simulink model "zumo_plant_custom_heading_original"  (R2014b)
settings: Solver=ode3  SolverMode=SingleTasking  StartTime=0.0  StopTime=2  FixedStep=0.01  RelTol=1e-3
PreLoadFcn:
  | evalin('base','sim=1;');
  | prepareCurrentFolderForZumo;
  | load MagnetometerBus;
model workspace (MAT data in the model file):
  axleLength = Simulink.Parameter
  axleLength.Value = 9.8
  axleLength.Description = 'Distance between tire contact points
    | of the two wheels/treads
    | in units of centimeters.'
  axleLength.DataType = 'auto'
  commandPercmPerSecond = Simulink.Parameter
  commandPercmPerSecond.Value = 3.9547
  commandPercmPerSecond.Description = 'Convert units of ''command'' 
    | to units of ''cm/s''.
    | 
    | ''command'' is a value in the range [-256, 255].'
  commandPercmPerSecond.DataType = 'auto'
  symmetrizeMotors = Simulink.Parameter
  symmetrizeMotors.Value = 1
  symmetrizeMotors.Description = 'Scale one of the motor commands down 
    | (not up) to balance the motors. 
    | Once balanced, a value of x sent to either
    | motor will produce the same rate of rotation
    | in both motors.'
  symmetrizeMotors.DataType = 'auto'
  sampleTime = Simulink.Parameter
  sampleTime.Value = 0.01
  sampleTime.Description = 'Sample time (in seconds) of the trajectory simulator.'
  sampleTime.DataType = 'auto'
  commandThreshold = Simulink.Parameter
  commandThreshold.Value = 31.875
  commandThreshold.DataType = 'auto'
  lineThreshold = Simulink.Parameter
  lineThreshold.Value = 500
  lineThreshold.DataType = 'auto'
  velocity = Simulink.Parameter
  velocity.Value = 10
  velocity.Description = 'cm / s'
  velocity.DataType = 'auto'
  waveLength = Simulink.Parameter
  waveLength.Value = 8.6
  waveLength.Description = 'Units of cm.
    | 
    | The following condition must be satisfied: 
    | waveLength > 2*pi * velocity / sqrt(0.5 / sampleTime)
    | 
    | For reference,
    | robotLength = 8.6 cm
    | '
  waveLength.DataType = 'auto'
  compassBias = Simulink.Parameter
  compassBias.Value = 0
  compassBias.DataType = 'auto'
undefined symbols (not defined in the file or in its folder): magnitude
libraries: simulink x5, ZumoBotLib x2
settings Model: ExtModeTrigDuration=2  Creator=pkasseba  LastModifiedBy=sandip
settings OptimizationCC: OptimizeModelRefInitCode=on  LifeSpan=1
settings DebuggingCC: UnderspecifiedInitializationDetection=Classic  MergeDetectMultiDrivingBlocksExec=none  SolverPrmCheckMsg=none  StateNameClashWarn=warning
settings HardwareCC: ProdBitPerInt=16  ProdBitPerPointer=8  ProdIntDivRoundTo=Zero  ProdEndianess=LittleEndian  ProdWordSize=8  ProdHWDeviceType=Atmel->AVR
settings SFSimCC: SimParseCustomCode=off
settings RTWCC: SystemTargetFile=realtime.tlc  GenerateMakefile=off  TemplateMakefile=realtime.tmf  Description=Run on Target Hardware  RTWVerbose=off  ProcessScript=realtime_make_rtw_hook
settings STFCustomTargetCC: TargetLibSuffix=.a  GenerateSampleERTMain=on  ERTCustomFileBanners=on  SupportNonInlinedSFcns=off  SupportVariableSizeSignals=on  MATLABClassNameForMDSCustomization=Simulink.SoftwareTarget.ERTCustomization  GRTInterface=off  SystemTargetFile=realtime.tlc
settings ERTTargetCC: GenerateSampleERTMain=on  ParMdlRefBuildCompliant=off  CompOptLevelCompliant=off  ConcurrentExecutionCompliant=off  CombineOutputUpdateFcns=off  ERTFirstTimeCompliant=off  SupportContinuousTime=on  SupportVariableSizeSignals=on  ModelStepFunctionPrototypeControlCompliant=off  CPPClassGenCompliant=off  ExtModeTransport=3  ExtModeMexFile=ext_serial_win32_comm  ExtModeMexArgs=0 1 9600  InlinedParameterPlacement=NonHierarchical  ERTSrcFileBannerTemplate=realtime_code_template.cgt  ERTHdrFileBannerTemplate=realtime_code_template.cgt  ERTDataSrcFileTemplate=realtime_code_template.cgt  ERTDataHdrFileTemplate=realtime_code_template.cgt  ERTCustomFileTemplate=realtime_file_process.tlc

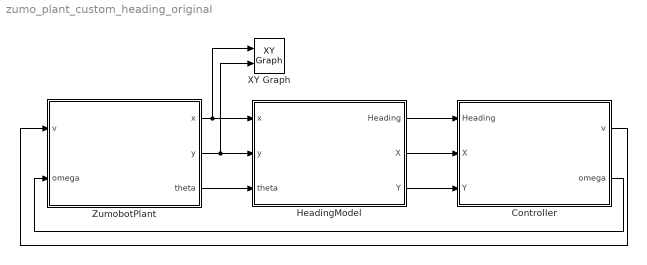
== system zumo_plant_custom_heading_original ==
  Controller : Subsystem
  HeadingModel : Subsystem  Variant=on
  XY Graph : simulink/Sinks/XY Graph  xmin=-10  xmax=50  ymin=-10  ymax=50  st=-1
  ZumobotPlant : Subsystem  Variant=on
  wires:
  Controller/1(v) -> ZumobotPlant/1(v)
  ZumobotPlant/1(x) -> XY Graph/1, HeadingModel/1(x)
  ZumobotPlant/2(y) -> XY Graph/2, HeadingModel/2(y)
  HeadingModel/1(Heading) -> Controller/1(Heading)
  Controller/2(omega) -> ZumobotPlant/2(omega)
  ZumobotPlant/3(theta) -> HeadingModel/3(theta)
  HeadingModel/2(X) -> Controller/2(X)
  HeadingModel/3(Y) -> Controller/3(Y)

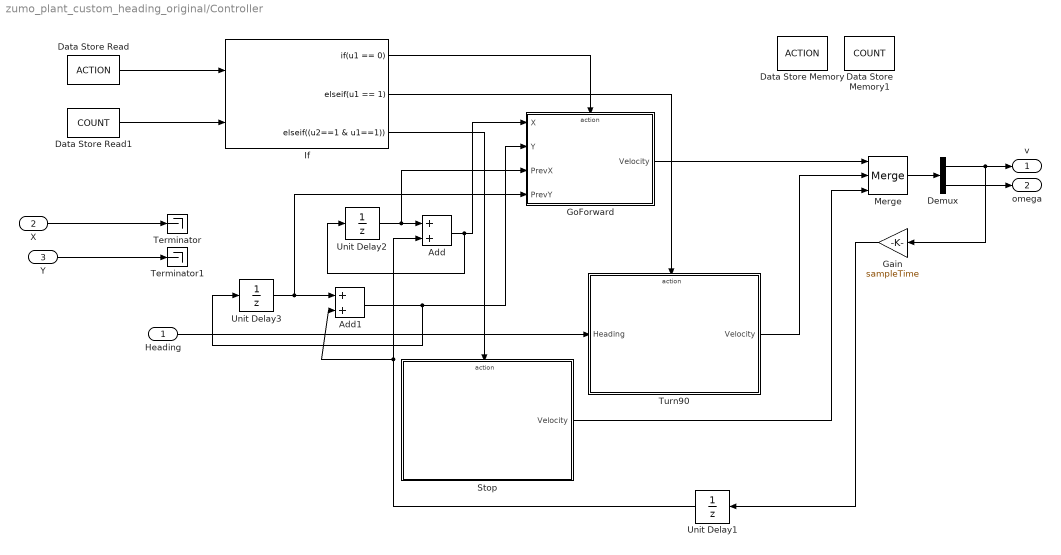
== system zumo_plant_custom_heading_original/Controller ==
  Heading : Inport
  X : Inport  Port=2
  Y : Inport  Port=3
  Add : Sum
  Add1 : Sum
  Data Store Memory : DataStoreMemory  DataStoreName=ACTION  ReadBeforeWriteMsg=warning  WriteAfterWriteMsg=warning  WriteAfterReadMsg=warning
  Data Store Memory1 : DataStoreMemory  DataStoreName=COUNT  ReadBeforeWriteMsg=warning  WriteAfterWriteMsg=warning  WriteAfterReadMsg=warning
  Data Store Read : DataStoreRead  DataStoreName=ACTION  SampleTime=sampleTime
  Data Store Read1 : DataStoreRead  DataStoreName=COUNT  SampleTime=sampleTime
  Demux : Demux  Outputs=2
  Gain : Gain  Gain=sampleTime
  GoForward : Subsystem  TreatAsAtomicUnit=on
  If : If  NumInputs=2  IfExpression=u1 == 0  ElseIfExpressions=u1 == 1, (u2==1 & u1==1)  ShowElse=off
  Merge : Merge  Inputs=3  InitialOutput=[0,0]
  Stop : Subsystem  TreatAsAtomicUnit=on
  Terminator : Terminator
  Terminator1 : Terminator
  Turn90 : Subsystem  TreatAsAtomicUnit=on
  Unit Delay1 : UnitDelay  SampleTime=-1
  Unit Delay2 : UnitDelay  SampleTime=-1
  Unit Delay3 : UnitDelay  SampleTime=-1
  v : Outport
  omega : Outport  Port=2
  wires:
  Demux/1 -> Gain/1, v/1
  Data Store Read/1 -> If/1
  If/1 -> GoForward/Action
  Heading/1 -> Turn90/1(Heading)
  If/2 -> Turn90/Action
  Data Store Read1/1 -> If/2
  If/3 -> Stop/Action
  GoForward/1(Velocity) -> Merge/1
  Turn90/1(Velocity) -> Merge/2
  Stop/1(Velocity) -> Merge/3
  Merge/1 -> Demux/1
  Demux/2 -> omega/1
  Gain/1 -> Unit Delay1/1
  Unit Delay2/1 -> GoForward/3(PrevX), Add/1
  Add/1 -> Unit Delay2/1, GoForward/1(X)
  Unit Delay3/1 -> GoForward/4(PrevY), Add1/1
  Add1/1 -> Unit Delay3/1, GoForward/2(Y)
  X/1 -> Terminator/1
  Y/1 -> Terminator1/1
  Unit Delay1/1 -> Add1/2, Add/2

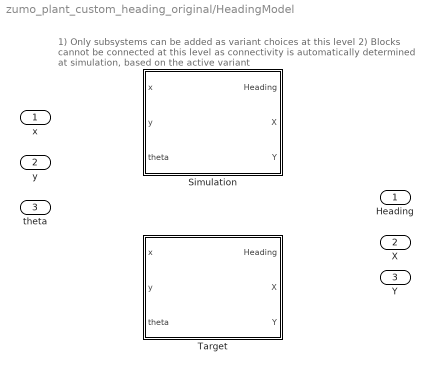
== system zumo_plant_custom_heading_original/HeadingModel ==
  note: 1) Only subsystems can be added as variant choices at this level
      | 2) Blocks cannot be connected at this level as connectivity is
      | automatically determined at simulation, based on the active variant
  x : Inport
  y : Inport  Port=2
  theta : Inport  Port=3
  Simulation : Subsystem  VariantControl=sim==1
  Target : Subsystem  VariantControl=sim==0
  Heading : Outport
  X : Outport  Port=2
  Y : Outport  Port=3

== system zumo_plant_custom_heading_original/ZumobotPlant ==
  note: 1) Only subsystems can be added as variant choices at this level
      | 2) Blocks cannot be connected at this level as connectivity is
      | automatically determined at simulation, based on the active variant
  v : Inport
  omega : Inport  Port=2
  Simulation : Subsystem  VariantControl=sim==1
  Target : Subsystem  VariantControl=sim==0
  x : Outport
  y : Outport  Port=2
  theta : Outport  Port=3

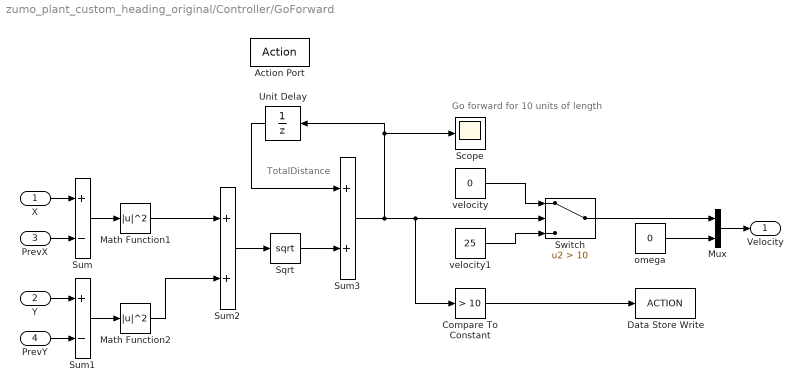
== system zumo_plant_custom_heading_original/Controller/GoForward ==
  note: Go forward for 10 units of length
  note: TotalDistance
  X : Inport
  Y : Inport  Port=2
  PrevX : Inport  Port=3
  PrevY : Inport  Port=4
  Action Port : ActionPort  InitializeStates=reset  ActionType=then
  Compare To Constant : simulink/Logic and Bit Operations/Compare To Constant  relop=>  const=10  OutDataTypeStr=boolean
  Data Store Write : DataStoreWrite  DataStoreName=ACTION
  Math Function1 : Math  Operator=magnitude^2  SaturateOnIntegerOverflow=on
  Math Function2 : Math  Operator=magnitude^2  SaturateOnIntegerOverflow=on
  Mux : Mux  Inputs=2
  Scope : Scope
      settings: YMin=0  YMax=50
  Sqrt : Sqrt  SaturateOnIntegerOverflow=on
  Sum : Sum  Inputs=+-
  Sum1 : Sum  Inputs=+-
  Sum2 : Sum
  Sum3 : Sum
  Switch : Switch  Criteria=u2 > Threshold  Threshold=10
  Unit Delay : UnitDelay  SampleTime=-1
  omega : Constant  Value=0
  velocity : Constant  Value=0
  velocity1 : Constant  Value=25
  Velocity : Outport  InitialOutput=[0 0]
  wires:
  X/1 -> Sum/1
  PrevX/1 -> Sum/2
  Y/1 -> Sum1/1
  PrevY/1 -> Sum1/2
  Sum/1 -> Math Function1/1
  Sum1/1 -> Math Function2/1
  Sum2/1 -> Sqrt/1
  Math Function2/1 -> Sum2/2
  Math Function1/1 -> Sum2/1
  Sqrt/1 -> Sum3/2
  Unit Delay/1 -> Sum3/1
  Mux/1 -> Velocity/1
  velocity/1 -> Switch/1
  velocity1/1 -> Switch/3
  Switch/1 -> Mux/1
  omega/1 -> Mux/2
  Compare To Constant/1 -> Data Store Write/1
  Sum3/1 -> Scope/1, Unit Delay/1, Compare To Constant/1, Switch/2

== system zumo_plant_custom_heading_original/Controller/Stop ==
  Action Port : ActionPort  InitializeStates=reset  ActionType=elseif
  Mux : Mux  Inputs=2
  omega : Constant  Value=0
  speed : Constant  Value=0
  Velocity : Outport  InitialOutput=[ 0 0 ]
  wires:
  Mux/1 -> Velocity/1
  speed/1 -> Mux/1
  omega/1 -> Mux/2

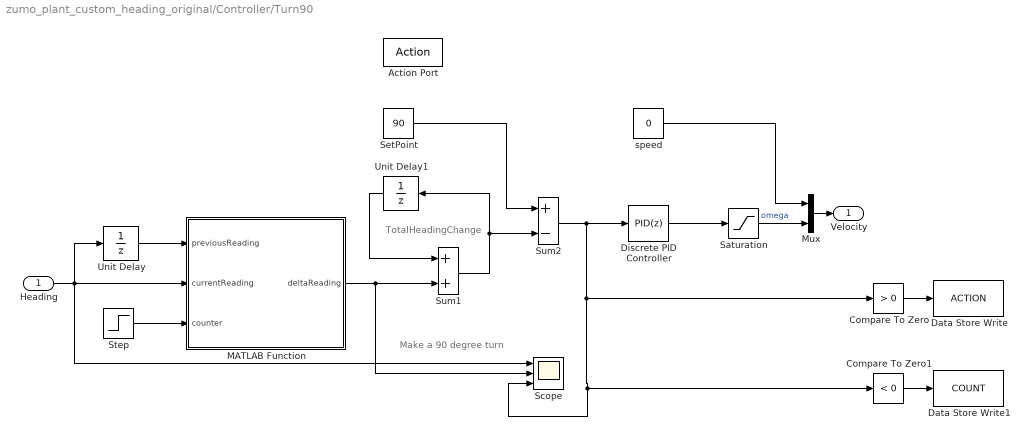
== system zumo_plant_custom_heading_original/Controller/Turn90 ==
  note: Make a 90 degree turn
  note: TotalHeadingChange
  Heading : Inport
  Action Port : ActionPort  InitializeStates=reset  ActionType=elseif
  Compare To Zero : simulink/Logic and Bit Operations/Compare To Zero  relop=>  OutDataTypeStr=boolean
  Compare To Zero1 : simulink/Logic and Bit Operations/Compare To Zero  relop=<  OutDataTypeStr=boolean
  Data Store Write : DataStoreWrite  DataStoreName=ACTION
  Data Store Write1 : DataStoreWrite  DataStoreName=COUNT
  Discrete PID Controller : simulink/Continuous/PID Controller  Controller=PID  TimeDomain=Discrete-time  SampleTime=0.01  IntegratorMethod=Forward Euler  FilterMethod=Forward Euler  Form=Parallel  P=100  I=0  D=0  N=100  InitialConditionSource=internal  InitialConditionForIntegrator=0  InitialConditionForFilter=0  ExternalReset=none  LimitOutput=off  UpperSaturationLimit=inf  LowerSaturationLimit=-inf  LinearizeAsGain=off  AntiWindupMode=none  Kb=1  TrackingMode=off  Kt=1  PParamMin=[]  PParamMax=[]  IParamMin=[]  IParamMax=[]  DParamMin=[]  DParamMax=[]  NParamMin=[]  NParamMax=[]  KbParamMin=[]  KbParamMax=[]  KtParamMin=[]  KtParamMax=[]  POutMin=[]  POutMax=[]  IOutMin=[]  IOutMax=[]  DOutMin=[]  DOutMax=[]  NOutMin=[]  NOutMax=[]  KbOutMin=[]  KbOutMax=[]  KtOutMin=[]  KtOutMax=[]  IntegratorOutMin=[]  IntegratorOutMax=[]  FilterOutMin=[]  FilterOutMax=[]  SumOutMin=[]  SumOutMax=[]  SumI1OutMin=[]  SumI1OutMax=[]  SumI2OutMin=[]  SumI2OutMax=[]  SumI3OutMin=[]  SumI3OutMax=[]  SumDOutMin=[]  SumDOutMax=[]  SaturationOutMin=[]  SaturationOutMax=[]  IntegratorContinuousStateAttributes=''  IntegratorStateMustResolveToSignalObject=off  IntegratorRTWStateStorageClass=Auto  FilterContinuousStateAttributes=''  FilterStateMustResolveToSignalObject=off  FilterRTWStateStorageClass=Auto  DifferentiatorICPrevScaledInput=0  DifferentiatorOutMin=[]  DifferentiatorOutMax=[]  UseFilter=on
  MATLAB Function : MATLAB Function  TreatAsAtomicUnit=on
  Mux : Mux  Inputs=2
  Saturation : Saturate  UpperLimit=200  LowerLimit=0
  Scope : Scope  NumInputPorts=3
      settings: YMin=252.7~-1~-4.2  YMax=279.3~1~-3.8
  SetPoint : Constant  Value=90
  Step : Step  Time=2*sampleTime  SampleTime=sampleTime
  Sum1 : Sum
  Sum2 : Sum  Inputs=+-
  Unit Delay : UnitDelay  SampleTime=-1
  Unit Delay1 : UnitDelay  SampleTime=-1
  speed : Constant  Value=0
  Velocity : Outport  InitialOutput=[0 0]
  wires:
  Sum2/1 -> Discrete PID Controller/1, Scope/3, Compare To Zero1/1, Compare To Zero/1
  Saturation/1 -> Mux/2  "omega"
  Sum1/1 -> Unit Delay1/1, Sum2/2
  MATLAB Function/1(deltaReading) -> Scope/2, Sum1/2
  SetPoint/1 -> Sum2/1
  Step/1 -> MATLAB Function/3(counter)
  Unit Delay/1 -> MATLAB Function/1(previousReading)
  Heading/1 -> Unit Delay/1, MATLAB Function/2(currentReading), Scope/1
  Unit Delay1/1 -> Sum1/1
  Mux/1 -> Velocity/1
  speed/1 -> Mux/1
  Compare To Zero/1 -> Data Store Write/1
  Compare To Zero1/1 -> Data Store Write1/1
  Discrete PID Controller/1 -> Saturation/1

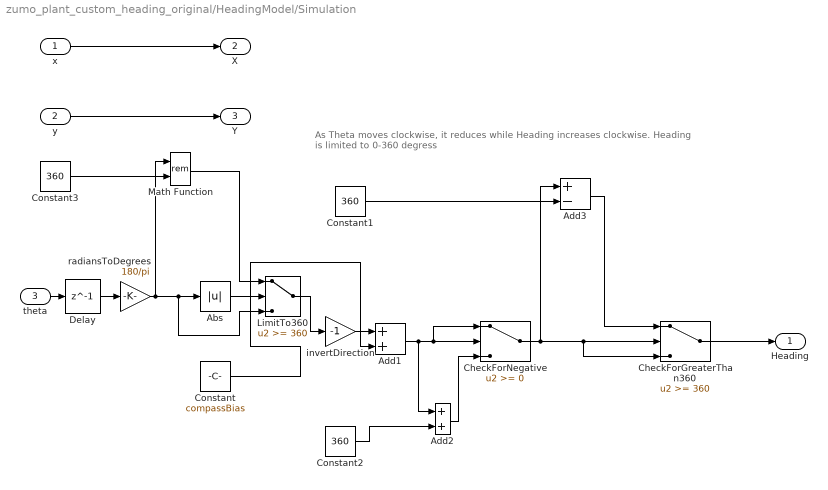
== system zumo_plant_custom_heading_original/HeadingModel/Simulation ==
  note: As Theta moves clockwise, it reduces while Heading increases clockwise.
      | Heading is limited to 0-360 degress
  x : Inport
  y : Inport  Port=2
  theta : Inport  Port=3
  Abs : Abs
  Add1 : Sum
  Add2 : Sum
  Add3 : Sum  Inputs=+-
  CheckForGreaterThan360 : Switch  Threshold=360
  CheckForNegative : Switch
  Constant : Constant  Value=compassBias
  Constant1 : Constant  Value=360
  Constant2 : Constant  Value=360
  Constant3 : Constant  Value=360
  Delay : Delay  DelayLength=1  InitialCondition=2*pi  SampleTime=sampleTime
  LimitTo360 : Switch  Threshold=360
  Math Function : Math  Operator=rem  SaturateOnIntegerOverflow=on
  invertDirection : Gain  Gain=-1
  radiansToDegrees : Gain  Gain=180/pi
  Heading : Outport
  X : Outport  Port=2
  Y : Outport  Port=3
  wires:
  x/1 -> X/1
  y/1 -> Y/1
  theta/1 -> Delay/1
  Delay/1 -> radiansToDegrees/1
  Constant/1 -> Add1/2
  Constant1/1 -> Add3/2
  CheckForGreaterThan360/1 -> Heading/1
  Add3/1 -> CheckForGreaterThan360/1
  invertDirection/1 -> Add1/1
  Add1/1 -> Add2/1, CheckForNegative/2, CheckForNegative/1
  CheckForNegative/1 -> CheckForGreaterThan360/3, CheckForGreaterThan360/2, Add3/1
  Constant2/1 -> Add2/2
  Add2/1 -> CheckForNegative/3
  radiansToDegrees/1 -> Math Function/1, LimitTo360/3, Abs/1
  LimitTo360/1 -> invertDirection/1
  Constant3/1 -> Math Function/2
  Math Function/1 -> LimitTo360/1
  Abs/1 -> LimitTo360/2

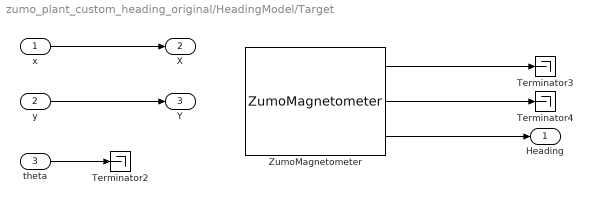
== system zumo_plant_custom_heading_original/HeadingModel/Target ==
  x : Inport
  y : Inport  Port=2
  theta : Inport  Port=3
  Terminator2 : Terminator
  Terminator3 : Terminator
  Terminator4 : Terminator
  ZumoMagnetometer : ZumoBotLib/ZumoMagnetometer  sampletime_lsm=0.01  debug_lsm=on  minX_lsm=-512  maxX_lsm=-279  minY_lsm=-163  maxY_lsm=99  minZ_lsm=1302  maxZ_lsm=1580
  Heading : Outport
  X : Outport  Port=2
  Y : Outport  Port=3
  wires:
  x/1 -> X/1
  y/1 -> Y/1
  theta/1 -> Terminator2/1
  ZumoMagnetometer/3 -> Heading/1
  ZumoMagnetometer/1 -> Terminator3/1
  ZumoMagnetometer/2 -> Terminator4/1

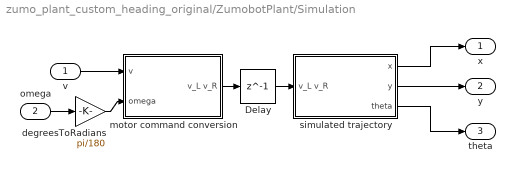
== system zumo_plant_custom_heading_original/ZumobotPlant/Simulation ==
  v : Inport
  omega : Inport  Port=2
  Delay : Delay  DelayLength=1  InitialCondition=0
  degreesToRadians : Gain  Gain=pi/180
  motor command conversion : Subsystem
  simulated trajectory : Subsystem
  x : Outport
  y : Outport  Port=2
  theta : Outport  Port=3
  wires:
  v/1 -> motor command conversion/1(v)
  simulated trajectory/1(x) -> x/1
  simulated trajectory/2(y) -> y/1
  omega/1 -> degreesToRadians/1
  simulated trajectory/3(theta) -> theta/1
  degreesToRadians/1 -> motor command conversion/2(omega)
  motor command conversion/1(v_L v_R) -> Delay/1
  Delay/1 -> simulated trajectory/1(v_L v_R)

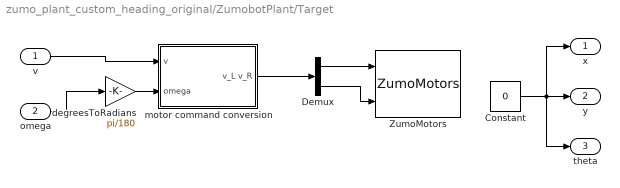
== system zumo_plant_custom_heading_original/ZumobotPlant/Target ==
  v : Inport
  omega : Inport  Port=2
  Constant : Constant  Value=0
  Demux : Demux  Outputs=2
  ZumoMotors : ZumoBotLib/ZumoMotors  flipLeft=off  flipRight=off
  degreesToRadians : Gain  Gain=pi/180
  motor command conversion : Subsystem
  x : Outport
  y : Outport  Port=2
  theta : Outport  Port=3
  wires:
  motor command conversion/1(v_L v_R) -> Demux/1
  Demux/1 -> ZumoMotors/1
  Demux/2 -> ZumoMotors/2
  v/1 -> motor command conversion/1(v)
  Constant/1 -> theta/1, x/1, y/1
  omega/1 -> degreesToRadians/1
  degreesToRadians/1 -> motor command conversion/2(omega)

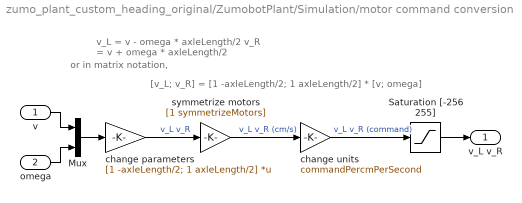
== system zumo_plant_custom_heading_original/ZumobotPlant/Simulation/motor command conversion ==
  note: or in matrix notation,
  note: v_L  = v - omega * axleLength/2
      | v_R = v + omega * axleLength/2
  note: [v_L; v_R] = [1 -axleLength/2; 1 axleLength/2] * [v; omega]
  v : Inport
  omega : Inport  Port=2
  Mux : Mux  Inputs=2
  Saturation [-256 255] : Saturate  UpperLimit=255  LowerLimit=-256
  change parameters : Gain  Gain=[1 -axleLength/2; 1 axleLength/2]  Multiplication=Matrix(K*u)
  change units : Gain  Gain=commandPercmPerSecond
  symmetrize motors : Gain  Gain=[1 symmetrizeMotors]
  v_L v_R : Outport
  wires:
  change parameters/1 -> symmetrize motors/1  "v_L v_R"
  change units/1 -> Saturation [-256 255]/1  "v_L v_R (command)"
  symmetrize motors/1 -> change units/1  "v_L v_R (cm/s)"
  Saturation [-256 255]/1 -> v_L v_R/1
  Mux/1 -> change parameters/1
  omega/1 -> Mux/2
  v/1 -> Mux/1

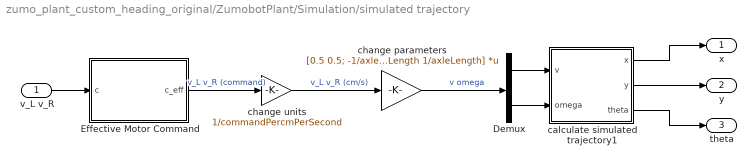
== system zumo_plant_custom_heading_original/ZumobotPlant/Simulation/simulated trajectory ==
  v_L v_R : Inport
  Demux : Demux  Outputs=2
  Effective Motor Command : Subsystem
  calculate simulated trajectory1 : Subsystem
  change parameters : Gain  Gain=[0.5 0.5; -1/axleLength 1/axleLength]  Multiplication=Matrix(K*u)
  change units : Gain  Gain=1/commandPercmPerSecond
  x : Outport
  y : Outport  Port=2
  theta : Outport  Port=3
  wires:
  Demux/2 -> calculate simulated trajectory1/2(omega)
  Demux/1 -> calculate simulated trajectory1/1(v)
  v_L v_R/1 -> Effective Motor Command/1(c)
  Effective Motor Command/1(c_eff) -> change units/1  "v_L v_R (command)"
  change units/1 -> change parameters/1  "v_L v_R (cm/s)"
  change parameters/1 -> Demux/1  "v omega"
  calculate simulated trajectory1/2(y) -> y/1
  calculate simulated trajectory1/3(theta) -> theta/1
  calculate simulated trajectory1/1(x) -> x/1

== system zumo_plant_custom_heading_original/ZumobotPlant/Target/motor command conversion ==
  note: or in matrix notation,
  note: v_L  = v - omega * axleLength/2
      | v_R = v + omega * axleLength/2
  note: [v_L; v_R] = [1 -axleLength/2; 1 axleLength/2] * [v; omega]
  v : Inport
  omega : Inport  Port=2
  Mux : Mux  Inputs=2
  Saturation [-256 255] : Saturate  UpperLimit=255  LowerLimit=-256
  change parameters : Gain  Gain=[1 -axleLength/2; 1 axleLength/2]  Multiplication=Matrix(K*u)
  change units : Gain  Gain=commandPercmPerSecond
  symmetrize motors : Gain  Gain=[1 symmetrizeMotors]
  v_L v_R : Outport
  wires:
  change parameters/1 -> symmetrize motors/1  "v_L v_R"
  change units/1 -> Saturation [-256 255]/1  "v_L v_R (command)"
  symmetrize motors/1 -> change units/1  "v_L v_R (cm/s)"
  Saturation [-256 255]/1 -> v_L v_R/1
  Mux/1 -> change parameters/1
  omega/1 -> Mux/2
  v/1 -> Mux/1

== system zumo_plant_custom_heading_original/ZumobotPlant/Simulation/simulated trajectory/Effective Motor Command ==
  note: Zumobot does not move when given a command
      | with an abs less than 50 on a smooth surface,
      | so such commands are effectively 0.
  note: Do not saturate this signal.The process of symmetrizing
      | the motor commands gives rise to this artificial signal,
      | which can exceed the value of 255.
  c : Inport
  Abs : Abs
  Constant1 : Constant  Value=0
  Sum : Sum  Inputs=|+-
  Switch : Switch
  command threshold : Constant  Value=commandThreshold
  symmetrize motors : Gain  Gain=[1 1/symmetrizeMotors]
  c_eff : Outport
  wires:
  Switch/1 -> c_eff/1
  symmetrize motors/1 -> Abs/1, Switch/1
  Sum/1 -> Switch/2
  Abs/1 -> Sum/1
  command threshold/1 -> Sum/2
  c/1 -> symmetrize motors/1  "v_L v_R"
  Constant1/1 -> Switch/3

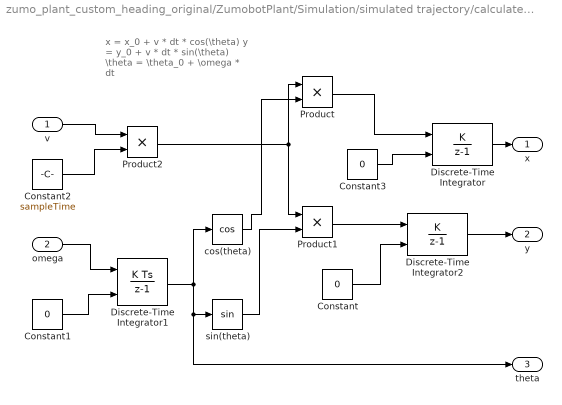
== system zumo_plant_custom_heading_original/ZumobotPlant/Simulation/simulated trajectory/calculate simulated trajectory1 ==
  note: x = x_0 + v * dt * cos(\theta)
      | y = y_0 + v * dt * sin(\theta)
      | \theta = \theta_0 + \omega * dt
  v : Inport
  omega : Inport  Port=2
  Constant : Constant  Value=0
  Constant1 : Constant  Value=0
  Constant2 : Constant  Value=sampleTime
  Constant3 : Constant  Value=0
  Discrete-Time Integrator : DiscreteIntegrator  IntegratorMethod=Accumulation: Forward Euler  InitialConditionSource=external  InitialConditionSetting=State (most efficient)  SampleTime=-1
  Discrete-Time Integrator1 : DiscreteIntegrator  InitialConditionSource=external  SampleTime=-1
  Discrete-Time Integrator2 : DiscreteIntegrator  IntegratorMethod=Accumulation: Forward Euler  InitialConditionSource=external  InitialConditionSetting=State (most efficient)  SampleTime=-1
  Product : Product
  Product1 : Product
  Product2 : Product
  cos(theta) : Trigonometry  Operator=cos
  sin(theta) : Trigonometry
  x : Outport
  y : Outport  Port=2
  theta : Outport  Port=3
  wires:
  omega/1 -> Discrete-Time Integrator1/1
  v/1 -> Product2/1
  Discrete-Time Integrator1/1 -> theta/1, sin(theta)/1, cos(theta)/1
  Product/1 -> Discrete-Time Integrator/1
  cos(theta)/1 -> Product/2
  Product2/1 -> Product/1, Product1/1
  sin(theta)/1 -> Product1/2
  Constant3/1 -> Discrete-Time Integrator/2
  Constant1/1 -> Discrete-Time Integrator1/2
  Constant2/1 -> Product2/2
  Discrete-Time Integrator/1 -> x/1
  Product1/1 -> Discrete-Time Integrator2/1
  Discrete-Time Integrator2/1 -> y/1
  Constant/1 -> Discrete-Time Integrator2/2

== matlab function zumo_plant_custom_heading_original/Controller/Turn90/MATLAB Function ==
  data: previousReading input; deltaReading output; currentReading input; counter input
function deltaReading = handle360jump(previousReading, currentReading, counter)
%#codegen
deltaReading = 0;
if counter
    deltaReading = currentReading - previousReading;
    if abs(deltaReading) > 300
        if deltaReading > 0
            deltaReading = 360 - currentReading + previousReading;
        else
            deltaReading = 360 + deltaReading;
        end
    end
end
deltaReading = abs(deltaReading);
